simulink model "case9"  (R2024b)
settings: Solver=FixedStepAuto  StartTime=0  StopTime=1  FixedStep=1e-7  RelTol=1e-3
values from neighbouring files (symbols this model uses):
  SG_D_1_D = 0.01056    [IEEE9_case_parameters.m]    (also in case1_parameters.m; case2_parameters.m; case3_parameters.m; case4_parameters.m)
  SG_D_1_EnableSaturation = 0    [IEEE9_case_parameters.m]    (also in case1_parameters.m; case2_parameters.m; case3_parameters.m; case4_parameters.m)
  SG_D_1_f0 = 60    [IEEE9_case_parameters.m]    (also in case1_parameters.m; case2_parameters.m; case3_parameters.m; case4_parameters.m)
  SG_D_1_H = 7.5    [IEEE9_case_parameters.m]    (also in case1_parameters.m; case2_parameters.m; case3_parameters.m; case4_parameters.m)
  SG_D_1_K_A = 20    [IEEE9_case_parameters.m]    (also in case1_parameters.m; case2_parameters.m; case3_parameters.m; case4_parameters.m)
  SG_D_1_K_E = 1.000000e+1    (= 10)    [IEEE9_case_parameters.m]    (also in case1_parameters.m; case2_parameters.m; case3_parameters.m; case4_parameters.m)
  SG_D_1_K_F = 2.363    [IEEE9_case_parameters.m]    (also in case1_parameters.m; case2_parameters.m; case3_parameters.m; case4_parameters.m)
  SG_D_1_K_s = 0.5    [IEEE9_case_parameters.m]    (also in case1_parameters.m = 5; case2_parameters.m = 5; case3_parameters.m = 5; case4_parameters.m = 5)
  SG_D_1_R_a = 0.001088    [IEEE9_case_parameters.m]    (also in case1_parameters.m; case2_parameters.m; case3_parameters.m; case4_parameters.m)
  SG_D_1_S_A = 1    [IEEE9_case_parameters.m]    (also in case1_parameters.m; case2_parameters.m; case3_parameters.m; case4_parameters.m)
  SG_D_1_S_B = 0.103    [IEEE9_case_parameters.m]    (also in case1_parameters.m; case2_parameters.m; case3_parameters.m; case4_parameters.m)
  SG_D_1_S_N = 10.659857    [IEEE9_case_parameters.m]    (also in case1_parameters.m; case2_parameters.m; case3_parameters.m; case4_parameters.m)
  SG_D_1_SpeedPara = 200    [IEEE9_case_parameters.m]    (also in case1_parameters.m; case2_parameters.m; case3_parameters.m; case4_parameters.m)
  SG_D_1_T_0 = 0.720173    [IEEE9_case_parameters.m]    (also in case1_parameters.m = 0.755522; case2_parameters.m = 0.808931; case3_parameters.m = 0.869402; case4_parameters.m = 0.729316)
  SG_D_1_T_1 = 0.3    [IEEE9_case_parameters.m]    (also in case1_parameters.m; case2_parameters.m; case3_parameters.m; case4_parameters.m)
  SG_D_1_T_2 = 0.05    [IEEE9_case_parameters.m]    (also in case1_parameters.m; case2_parameters.m; case3_parameters.m; case4_parameters.m)
  SG_D_1_T_3 = 0.02    [IEEE9_case_parameters.m]    (also in case1_parameters.m; case2_parameters.m; case3_parameters.m; case4_parameters.m)
  SG_D_1_T_4 = 0.005    [IEEE9_case_parameters.m]    (also in case1_parameters.m; case2_parameters.m; case3_parameters.m; case4_parameters.m)
  SG_D_1_T_A = 0.02    [IEEE9_case_parameters.m]    (also in case1_parameters.m; case2_parameters.m; case3_parameters.m; case4_parameters.m)
  SG_D_1_T_dd = 8.000000e+0    (= 8)    [IEEE9_case_parameters.m]    (also in case1_parameters.m; case2_parameters.m; case3_parameters.m; case4_parameters.m)
  SG_D_1_T_ddd = 0.04    [IEEE9_case_parameters.m]    (also in case1_parameters.m; case2_parameters.m; case3_parameters.m; case4_parameters.m)
  SG_D_1_T_E = 0.314    [IEEE9_case_parameters.m]    (also in case1_parameters.m; case2_parameters.m; case3_parameters.m; case4_parameters.m)
  SG_D_1_T_F = 0.35    [IEEE9_case_parameters.m]    (also in case1_parameters.m; case2_parameters.m; case3_parameters.m; case4_parameters.m)
  SG_D_1_T_qd = 0.8    [IEEE9_case_parameters.m]    (also in case1_parameters.m; case2_parameters.m; case3_parameters.m; case4_parameters.m)
  SG_D_1_T_qdd = 0.02    [IEEE9_case_parameters.m]    (also in case1_parameters.m; case2_parameters.m; case3_parameters.m; case4_parameters.m)
  SG_D_1_T_speed = 0.1    [IEEE9_case_parameters.m]    (also in case1_parameters.m = 200; case2_parameters.m = 200; case3_parameters.m = 200; case4_parameters.m = 200)
  SG_D_1_T_w = 0.5    [IEEE9_case_parameters.m]    (also in case1_parameters.m; case2_parameters.m; case3_parameters.m; case4_parameters.m)
  SG_D_1_V_ref = 1.990276    [IEEE9_case_parameters.m]    (also in case1_parameters.m = 2.042296; case2_parameters.m = 2.051388; case3_parameters.m = 2.089584; case4_parameters.m = 2.01845)
  SG_D_1_w_ref = 376.991118    [IEEE9_case_parameters.m]    (also in case1_parameters.m; case2_parameters.m; case3_parameters.m; case4_parameters.m)
  SG_D_1_wb = 6.000000e+1    (= 60)    [IEEE9_case_parameters.m]    (also in case1_parameters.m; case2_parameters.m; case3_parameters.m; case4_parameters.m)
  SG_D_1_x_d = 1.9    [IEEE9_case_parameters.m]    (also in case1_parameters.m; case2_parameters.m; case3_parameters.m; case4_parameters.m)
  SG_D_1_x_dd = 0.302    [IEEE9_case_parameters.m]    (also in case1_parameters.m; case2_parameters.m; case3_parameters.m; case4_parameters.m)
  SG_D_1_x_ddd = 0.204    [IEEE9_case_parameters.m]    (also in case1_parameters.m; case2_parameters.m; case3_parameters.m; case4_parameters.m)
  SG_D_1_x_l = 0.05    [IEEE9_case_parameters.m]    (also in case1_parameters.m; case2_parameters.m; case3_parameters.m; case4_parameters.m)
  SG_D_1_x_q = 1.3    [IEEE9_case_parameters.m]    (also in case1_parameters.m; case2_parameters.m; case3_parameters.m; case4_parameters.m)
  SG_D_1_x_qd = 0.5    [IEEE9_case_parameters.m]    (also in case1_parameters.m; case2_parameters.m; case3_parameters.m; case4_parameters.m)
  SG_D_1_x_qdd = 0.3    [IEEE9_case_parameters.m]    (also in case1_parameters.m; case2_parameters.m; case3_parameters.m; case4_parameters.m)
  SG_D_2_D = 0.02    [IEEE9_case_parameters.m]    (also in case1_parameters.m; case2_parameters.m; case3_parameters.m; case4_parameters.m)
  SG_D_2_EnableSaturation = 0    [IEEE9_case_parameters.m]    (also in case1_parameters.m; case2_parameters.m; case3_parameters.m; case4_parameters.m)
  SG_D_2_f0 = 60    [IEEE9_case_parameters.m]    (also in case1_parameters.m; case2_parameters.m; case3_parameters.m; case4_parameters.m)
  SG_D_2_H = 8.000000e+0    (= 8)    [IEEE9_case_parameters.m]    (also in case1_parameters.m; case2_parameters.m; case3_parameters.m; case4_parameters.m)
  SG_D_2_K_A = 20    [IEEE9_case_parameters.m]    (also in case1_parameters.m; case2_parameters.m; case3_parameters.m; case4_parameters.m)
  SG_D_2_K_E = 1.000000e+1    (= 10)    [IEEE9_case_parameters.m]    (also in case1_parameters.m; case2_parameters.m; case3_parameters.m; case4_parameters.m)
  SG_D_2_K_F = 2.363    [IEEE9_case_parameters.m]    (also in case1_parameters.m; case2_parameters.m; case3_parameters.m; case4_parameters.m)
  SG_D_2_K_s = 0.5    [IEEE9_case_parameters.m]    (also in case1_parameters.m = 4; case2_parameters.m = 4; case3_parameters.m = 4; case4_parameters.m = 4)
  SG_D_2_R_a = 0.001088    [IEEE9_case_parameters.m]    (also in case1_parameters.m; case2_parameters.m; case3_parameters.m; case4_parameters.m)
  SG_D_2_S_A = 1    [IEEE9_case_parameters.m]    (also in case1_parameters.m; case2_parameters.m; case3_parameters.m; case4_parameters.m)
  SG_D_2_S_B = 0.103    [IEEE9_case_parameters.m]    (also in case1_parameters.m; case2_parameters.m; case3_parameters.m; case4_parameters.m)
  SG_D_2_S_N = 10.659857    [IEEE9_case_parameters.m]    (also in case1_parameters.m; case2_parameters.m; case3_parameters.m; case4_parameters.m)
  SG_D_2_SpeedPara = 200    [IEEE9_case_parameters.m]    (also in case1_parameters.m; case2_parameters.m; case3_parameters.m; case4_parameters.m)
  SG_D_2_T_0 = 1.632913    [IEEE9_case_parameters.m]    (also in case1_parameters.m = 1.632925; case2_parameters.m = 1.632915; case3_parameters.m = 1.632914; case4_parameters.m = 1.632927)
  SG_D_2_T_1 = 0.2    [IEEE9_case_parameters.m]    (also in case1_parameters.m; case2_parameters.m; case3_parameters.m; case4_parameters.m)
  SG_D_2_T_2 = 0.05    [IEEE9_case_parameters.m]    (also in case1_parameters.m; case2_parameters.m; case3_parameters.m; case4_parameters.m)
  SG_D_2_T_3 = 0.02    [IEEE9_case_parameters.m]    (also in case1_parameters.m; case2_parameters.m; case3_parameters.m; case4_parameters.m)
  SG_D_2_T_4 = 0.005    [IEEE9_case_parameters.m]    (also in case1_parameters.m; case2_parameters.m; case3_parameters.m; case4_parameters.m)
  SG_D_2_T_A = 0.02    [IEEE9_case_parameters.m]    (also in case1_parameters.m; case2_parameters.m; case3_parameters.m; case4_parameters.m)
  SG_D_2_T_dd = 7.9    [IEEE9_case_parameters.m]    (also in case1_parameters.m; case2_parameters.m; case3_parameters.m; case4_parameters.m)
  SG_D_2_T_ddd = 0.04    [IEEE9_case_parameters.m]    (also in case1_parameters.m; case2_parameters.m; case3_parameters.m; case4_parameters.m)
  SG_D_2_T_E = 0.314    [IEEE9_case_parameters.m]    (also in case1_parameters.m; case2_parameters.m; case3_parameters.m; case4_parameters.m)
  SG_D_2_T_F = 0.35    [IEEE9_case_parameters.m]    (also in case1_parameters.m; case2_parameters.m; case3_parameters.m; case4_parameters.m)
  SG_D_2_T_qd = 0.8    [IEEE9_case_parameters.m]    (also in case1_parameters.m; case2_parameters.m; case3_parameters.m; case4_parameters.m)
  SG_D_2_T_qdd = 0.015    [IEEE9_case_parameters.m]    (also in case1_parameters.m; case2_parameters.m; case3_parameters.m; case4_parameters.m)
  SG_D_2_T_speed = 0.1    [IEEE9_case_parameters.m]    (also in case1_parameters.m = 150; case2_parameters.m = 150; case3_parameters.m = 150; case4_parameters.m = 150)
  SG_D_2_T_w = 0.35    [IEEE9_case_parameters.m]    (also in case1_parameters.m; case2_parameters.m; case3_parameters.m; case4_parameters.m)
  SG_D_2_V_ref = 2.58547    [IEEE9_case_parameters.m]    (also in case1_parameters.m = 2.597896; case2_parameters.m = 2.587136; case3_parameters.m = 2.586042; case4_parameters.m = 2.599679)
  SG_D_2_w_ref = 376.991118    [IEEE9_case_parameters.m]    (also in case1_parameters.m; case2_parameters.m; case3_parameters.m; case4_parameters.m)
  SG_D_2_wb = 6.000000e+1    (= 60)    [IEEE9_case_parameters.m]    (also in case1_parameters.m; case2_parameters.m; case3_parameters.m; case4_parameters.m)
  SG_D_2_x_d = 1.8    [IEEE9_case_parameters.m]    (also in case1_parameters.m; case2_parameters.m; case3_parameters.m; case4_parameters.m)
  SG_D_2_x_dd = 0.302    [IEEE9_case_parameters.m]    (also in case1_parameters.m; case2_parameters.m; case3_parameters.m; case4_parameters.m)
  SG_D_2_x_ddd = 0.204    [IEEE9_case_parameters.m]    (also in case1_parameters.m; case2_parameters.m; case3_parameters.m; case4_parameters.m)
  SG_D_2_x_l = 0.05    [IEEE9_case_parameters.m]    (also in case1_parameters.m; case2_parameters.m; case3_parameters.m; case4_parameters.m)
  SG_D_2_x_q = 1.25    [IEEE9_case_parameters.m]    (also in case1_parameters.m; case2_parameters.m; case3_parameters.m; case4_parameters.m)
  SG_D_2_x_qd = 0.5    [IEEE9_case_parameters.m]    (also in case1_parameters.m; case2_parameters.m; case3_parameters.m; case4_parameters.m)
  SG_D_2_x_qdd = 0.3    [IEEE9_case_parameters.m]    (also in case1_parameters.m; case2_parameters.m; case3_parameters.m; case4_parameters.m)
  SG_D_3_D = 0.02    [IEEE9_case_parameters.m]    (also in case1_parameters.m; case2_parameters.m; case3_parameters.m; case4_parameters.m)
  SG_D_3_EnableSaturation = 0    [IEEE9_case_parameters.m]    (also in case1_parameters.m; case2_parameters.m; case3_parameters.m; case4_parameters.m)
  SG_D_3_f0 = 60    [IEEE9_case_parameters.m]    (also in case1_parameters.m; case2_parameters.m; case3_parameters.m; case4_parameters.m)
  SG_D_3_H = 7.7    [IEEE9_case_parameters.m]    (also in case1_parameters.m; case2_parameters.m; case3_parameters.m; case4_parameters.m)
  SG_D_3_K_A = 20    [IEEE9_case_parameters.m]    (also in case1_parameters.m; case2_parameters.m; case3_parameters.m; case4_parameters.m)
  SG_D_3_K_E = 1.000000e+1    (= 10)    [IEEE9_case_parameters.m]    (also in case1_parameters.m; case2_parameters.m; case3_parameters.m; case4_parameters.m)
  SG_D_3_K_F = 2.363    [IEEE9_case_parameters.m]    (also in case1_parameters.m; case2_parameters.m; case3_parameters.m; case4_parameters.m)
  SG_D_3_K_s = 0.2    [IEEE9_case_parameters.m]    (also in case1_parameters.m = 2; case2_parameters.m = 2; case3_parameters.m = 2; case4_parameters.m = 2)
  SG_D_3_R_a = 0.001088    [IEEE9_case_parameters.m]    (also in case1_parameters.m; case2_parameters.m; case3_parameters.m; case4_parameters.m)
  SG_D_3_S_A = 1    [IEEE9_case_parameters.m]    (also in case1_parameters.m; case2_parameters.m; case3_parameters.m; case4_parameters.m)
  SG_D_3_S_B = 0.103    [IEEE9_case_parameters.m]    (also in case1_parameters.m; case2_parameters.m; case3_parameters.m; case4_parameters.m)
  SG_D_3_S_N = 10.659857    [IEEE9_case_parameters.m]    (also in case1_parameters.m; case2_parameters.m; case3_parameters.m; case4_parameters.m)
  SG_D_3_SpeedPara = 200    [IEEE9_case_parameters.m]    (also in case1_parameters.m; case2_parameters.m; case3_parameters.m; case4_parameters.m)
  SG_D_3_T_0 = 0.850788    [IEEE9_case_parameters.m]    (also in case1_parameters.m = 0.850786; case2_parameters.m = 0.850787; case3_parameters.m; case4_parameters.m = 0.850786)
  SG_D_3_T_1 = 0.2    [IEEE9_case_parameters.m]    (also in case1_parameters.m; case2_parameters.m; case3_parameters.m; case4_parameters.m)
  SG_D_3_T_2 = 0.05    [IEEE9_case_parameters.m]    (also in case1_parameters.m; case2_parameters.m; case3_parameters.m; case4_parameters.m)
  SG_D_3_T_3 = 0.02    [IEEE9_case_parameters.m]    (also in case1_parameters.m; case2_parameters.m; case3_parameters.m; case4_parameters.m)
  SG_D_3_T_4 = 0.005    [IEEE9_case_parameters.m]    (also in case1_parameters.m; case2_parameters.m; case3_parameters.m; case4_parameters.m)
  SG_D_3_T_A = 0.02    [IEEE9_case_parameters.m]    (also in case1_parameters.m; case2_parameters.m; case3_parameters.m; case4_parameters.m)
  SG_D_3_T_dd = 8.1    [IEEE9_case_parameters.m]    (also in case1_parameters.m; case2_parameters.m; case3_parameters.m; case4_parameters.m)
  SG_D_3_T_ddd = 0.04    [IEEE9_case_parameters.m]    (also in case1_parameters.m; case2_parameters.m; case3_parameters.m; case4_parameters.m)
  SG_D_3_T_E = 0.314    [IEEE9_case_parameters.m]    (also in case1_parameters.m; case2_parameters.m; case3_parameters.m; case4_parameters.m)
  SG_D_3_T_F = 0.35    [IEEE9_case_parameters.m]    (also in case1_parameters.m; case2_parameters.m; case3_parameters.m; case4_parameters.m)
  SG_D_3_T_qd = 0.8    [IEEE9_case_parameters.m]    (also in case1_parameters.m; case2_parameters.m; case3_parameters.m; case4_parameters.m)
  SG_D_3_T_qdd = 0.015    [IEEE9_case_parameters.m]    (also in case1_parameters.m; case2_parameters.m; case3_parameters.m; case4_parameters.m)
  SG_D_3_T_speed = 0.1    [IEEE9_case_parameters.m]    (also in case1_parameters.m = 180; case2_parameters.m = 180; case3_parameters.m = 180; case4_parameters.m = 180)
  SG_D_3_T_w = 0.4    [IEEE9_case_parameters.m]    (also in case1_parameters.m; case2_parameters.m; case3_parameters.m; case4_parameters.m)
  SG_D_3_V_ref = 1.892727    [IEEE9_case_parameters.m]    (also in case1_parameters.m = 1.906439; case2_parameters.m = 1.895535; case3_parameters.m = 1.892105; case4_parameters.m = 1.906598)
  SG_D_3_w_ref = 376.991118    [IEEE9_case_parameters.m]    (also in case1_parameters.m; case2_parameters.m; case3_parameters.m; case4_parameters.m)
  SG_D_3_wb = 6.000000e+1    (= 60)    [IEEE9_case_parameters.m]    (also in case1_parameters.m; case2_parameters.m; case3_parameters.m; case4_parameters.m)
  SG_D_3_x_d = 1.85    [IEEE9_case_parameters.m]    (also in case1_parameters.m; case2_parameters.m; case3_parameters.m; case4_parameters.m)
  SG_D_3_x_dd = 0.302    [IEEE9_case_parameters.m]    (also in case1_parameters.m; case2_parameters.m; case3_parameters.m; case4_parameters.m)
  SG_D_3_x_ddd = 0.204    [IEEE9_case_parameters.m]    (also in case1_parameters.m; case2_parameters.m; case3_parameters.m; case4_parameters.m)
  SG_D_3_x_l = 0.05    [IEEE9_case_parameters.m]    (also in case1_parameters.m; case2_parameters.m; case3_parameters.m; case4_parameters.m)
  SG_D_3_x_q = 1.2    [IEEE9_case_parameters.m]    (also in case1_parameters.m; case2_parameters.m; case3_parameters.m; case4_parameters.m)
  SG_D_3_x_qd = 0.5    [IEEE9_case_parameters.m]    (also in case1_parameters.m; case2_parameters.m; case3_parameters.m; case4_parameters.m)
  SG_D_3_x_qdd = 0.3    [IEEE9_case_parameters.m]    (also in case1_parameters.m; case2_parameters.m; case3_parameters.m; case4_parameters.m)
(part 3 of 12)

== system case9/AC_1/d_vq_bus_2_block ==
  note: d_vq_bus_2 in case9
      | $37699111.8430775\,\mathrm{iq}_{\mathrm{bus},2}-376.991118430775\,\mathrm{vd}_{\mathrm{bus},2}$
      | Automatically generated on 2025-10-31 19:35:33 .
  Alge_iq_bus_2_77b03 : Inport
  State_vd_bus_2_31c31 : Inport  Port=2
  Constant_376.991118430775_297b4 : Constant  Value=376.991118430775
  Constant_37699111.8430775_23c38 : Constant  Value=37699111.8430775
  Product_78845 : Product
  Product_c8408 : Product
  Subtract_e18ad : Sum  Inputs=+-
  Blockout_d_vq_bus_2_4c26a : Outport
  wires:
  Constant_37699111.8430775_23c38/1 -> Product_78845/1
  Constant_376.991118430775_297b4/1 -> Product_c8408/1
  Alge_iq_bus_2_77b03/1 -> Product_78845/2
  State_vd_bus_2_31c31/1 -> Product_c8408/2
  Product_78845/1 -> Subtract_e18ad/1
  Product_c8408/1 -> Subtract_e18ad/2
  Subtract_e18ad/1 -> Blockout_d_vq_bus_2_4c26a/1

== system case9/AC_1/d_vq_bus_3_block ==
  note: d_vq_bus_3 in case9
      | $37699111.8430775\,\mathrm{iq}_{\mathrm{bus},3}-376.991118430775\,\mathrm{vd}_{\mathrm{bus},3}$
      | Automatically generated on 2025-10-31 19:35:34 .
  Alge_iq_bus_3_cc23e : Inport
  State_vd_bus_3_6cfca : Inport  Port=2
  Constant_376.991118430775_aad21 : Constant  Value=376.991118430775
  Constant_37699111.8430775_489f0 : Constant  Value=37699111.8430775
  Product_2d405 : Product
  Product_442e1 : Product
  Subtract_58085 : Sum  Inputs=+-
  Blockout_d_vq_bus_3_a4433 : Outport
  wires:
  Constant_37699111.8430775_489f0/1 -> Product_2d405/1
  Constant_376.991118430775_aad21/1 -> Product_442e1/1
  Alge_iq_bus_3_cc23e/1 -> Product_2d405/2
  State_vd_bus_3_6cfca/1 -> Product_442e1/2
  Product_2d405/1 -> Subtract_58085/1
  Product_442e1/1 -> Subtract_58085/2
  Subtract_58085/1 -> Blockout_d_vq_bus_3_a4433/1

== system case9/AC_1/d_vq_bus_4_block ==
  note: d_vq_bus_4 in case9
      | $2257.43184689087\,\mathrm{iq}_{\mathrm{bus},4}-376.991118430775\,\mathrm{vd}_{\mathrm{bus},4}$
      | Automatically generated on 2025-10-31 19:35:34 .
  Alge_iq_bus_4_57fc4 : Inport
  State_vd_bus_4_4807b : Inport  Port=2
  Constant_2257.43184689087_35413 : Constant  Value=2257.43184689087
  Constant_376.991118430775_cfbfc : Constant  Value=376.991118430775
  Product_cb25e : Product
  Product_f6559 : Product
  Subtract_ca4f2 : Sum  Inputs=+-
  Blockout_d_vq_bus_4_b4e62 : Outport
  wires:
  Constant_2257.43184689087_35413/1 -> Product_f6559/1
  Constant_376.991118430775_cfbfc/1 -> Product_cb25e/1
  Alge_iq_bus_4_57fc4/1 -> Product_f6559/2
  State_vd_bus_4_4807b/1 -> Product_cb25e/2
  Product_f6559/1 -> Subtract_ca4f2/1
  Product_cb25e/1 -> Subtract_ca4f2/2
  Subtract_ca4f2/1 -> Blockout_d_vq_bus_4_b4e62/1

== system case9/AC_1/d_vq_bus_5_block ==
  note: d_vq_bus_5 in case9
      | $1461.2058853906\,\mathrm{iq}_{\mathrm{bus},5}-376.991118430775\,\mathrm{vd}_{\mathrm{bus},5}$
      | Automatically generated on 2025-10-31 19:35:35 .
  Alge_iq_bus_5_8c66c : Inport
  State_vd_bus_5_846f7 : Inport  Port=2
  Constant_1461.2058853906_0d7a9 : Constant  Value=1461.2058853906
  Constant_376.991118430775_e6df8 : Constant  Value=376.991118430775
  Product_c1e2f : Product
  Product_fd608 : Product
  Subtract_c2c85 : Sum  Inputs=+-
  Blockout_d_vq_bus_5_0bbb7 : Outport
  wires:
  Constant_1461.2058853906_0d7a9/1 -> Product_fd608/1
  Constant_376.991118430775_e6df8/1 -> Product_c1e2f/1
  Alge_iq_bus_5_8c66c/1 -> Product_fd608/2
  State_vd_bus_5_846f7/1 -> Product_c1e2f/2
  Product_fd608/1 -> Subtract_c2c85/1
  Product_c1e2f/1 -> Subtract_c2c85/2
  Subtract_c2c85/1 -> Blockout_d_vq_bus_5_0bbb7/1

== system case9/AC_1/d_vq_bus_6_block ==
  note: d_vq_bus_6 in case9
      | $1329.77466818616\,\mathrm{iq}_{\mathrm{bus},6}-376.991118430775\,\mathrm{vd}_{\mathrm{bus},6}$
      | Automatically generated on 2025-10-31 19:35:35 .
  Alge_iq_bus_6_d852c : Inport
  State_vd_bus_6_933d9 : Inport  Port=2
  Constant_1329.77466818616_4ee96 : Constant  Value=1329.77466818616
  Constant_376.991118430775_b81da : Constant  Value=376.991118430775
  Product_b7a54 : Product
  Product_c8743 : Product
  Subtract_aadba : Sum  Inputs=+-
  Blockout_d_vq_bus_6_9d5e1 : Outport
  wires:
  Constant_1329.77466818616_4ee96/1 -> Product_c8743/1
  Constant_376.991118430775_b81da/1 -> Product_b7a54/1
  Alge_iq_bus_6_d852c/1 -> Product_c8743/2
  State_vd_bus_6_933d9/1 -> Product_b7a54/2
  Product_c8743/1 -> Subtract_aadba/1
  Product_b7a54/1 -> Subtract_aadba/2
  Subtract_aadba/1 -> Blockout_d_vq_bus_6_9d5e1/1

== system case9/AC_1/d_vq_bus_7_block ==
  note: d_vq_bus_7 in case9
      | $2106.09563369148\,\mathrm{iq}_{\mathrm{bus},7}-376.991118430775\,\mathrm{vd}_{\mathrm{bus},7}$
      | Automatically generated on 2025-10-31 19:35:36 .
  Alge_iq_bus_7_10ac4 : Inport
  State_vd_bus_7_f1873 : Inport  Port=2
  Constant_2106.09563369148_b1513 : Constant  Value=2106.09563369148
  Constant_376.991118430775_e1123 : Constant  Value=376.991118430775
  Product_6b0d5 : Product
  Product_fc3db : Product
  Subtract_4ac9d : Sum  Inputs=+-
  Blockout_d_vq_bus_7_bd4da : Outport
  wires:
  Constant_2106.09563369148_b1513/1 -> Product_fc3db/1
  Product_6b0d5/1 -> Subtract_4ac9d/2
  Alge_iq_bus_7_10ac4/1 -> Product_fc3db/2
  Constant_376.991118430775_e1123/1 -> Product_6b0d5/1
  Subtract_4ac9d/1 -> Blockout_d_vq_bus_7_bd4da/1
  State_vd_bus_7_f1873/1 -> Product_6b0d5/2
  Product_fc3db/1 -> Subtract_4ac9d/1

== system case9/AC_1/d_vq_bus_8_block ==
  note: d_vq_bus_8 in case9
      | $1657.10381727813\,\mathrm{iq}_{\mathrm{bus},8}-376.991118430775\,\mathrm{vd}_{\mathrm{bus},8}$
      | Automatically generated on 2025-10-31 19:35:36 .
  Alge_iq_bus_8_70786 : Inport
  State_vd_bus_8_2f4e8 : Inport  Port=2
  Constant_1657.10381727813_470a7 : Constant  Value=1657.10381727813
  Constant_376.991118430775_75430 : Constant  Value=376.991118430775
  Product_04e24 : Product
  Product_0a383 : Product
  Subtract_4f591 : Sum  Inputs=+-
  Blockout_d_vq_bus_8_7a639 : Outport
  wires:
  Constant_1657.10381727813_470a7/1 -> Product_04e24/1
  Constant_376.991118430775_75430/1 -> Product_0a383/1
  Alge_iq_bus_8_70786/1 -> Product_04e24/2
  State_vd_bus_8_2f4e8/1 -> Product_0a383/2
  Product_04e24/1 -> Subtract_4f591/1
  Product_0a383/1 -> Subtract_4f591/2
  Subtract_4f591/1 -> Blockout_d_vq_bus_8_7a639/1

== system case9/AC_1/d_vq_bus_9_block ==
  note: d_vq_bus_9 in case9
      | $1564.27849971276\,\mathrm{iq}_{\mathrm{bus},9}-376.991118430775\,\mathrm{vd}_{\mathrm{bus},9}$
      | Automatically generated on 2025-10-31 19:35:37 .
  Alge_iq_bus_9_d89c6 : Inport
  State_vd_bus_9_9eb2e : Inport  Port=2
  Constant_1564.27849971276_ed724 : Constant  Value=1564.27849971276
  Constant_376.991118430775_3314c : Constant  Value=376.991118430775
  Product_29196 : Product
  Product_ab7b2 : Product
  Subtract_c7e30 : Sum  Inputs=+-
  Blockout_d_vq_bus_9_68009 : Outport
  wires:
  Constant_1564.27849971276_ed724/1 -> Product_29196/1
  Constant_376.991118430775_3314c/1 -> Product_ab7b2/1
  Alge_iq_bus_9_d89c6/1 -> Product_29196/2
  State_vd_bus_9_9eb2e/1 -> Product_ab7b2/2
  Product_29196/1 -> Subtract_c7e30/1
  Product_ab7b2/1 -> Subtract_c7e30/2
  Subtract_c7e30/1 -> Blockout_d_vq_bus_9_68009/1

== system case9/AC_1/id_bus_1_block ==
  note: id_bus_1 in case9
      | $\mathrm{id}_{\mathrm{SG},D,1}-\mathrm{id}_{\mathrm{line},1,4}$
      | Automatically generated on 2025-10-31 19:35:48 .
  Input_id_SG_D_1_08570 : Inport
  State_id_line_1_4_a7c42 : Inport  Port=2
  Subtract_91534 : Sum  Inputs=+-
  Blockout_id_bus_1_e658d : Outport
  wires:
  Input_id_SG_D_1_08570/1 -> Subtract_91534/1
  State_id_line_1_4_a7c42/1 -> Subtract_91534/2
  Subtract_91534/1 -> Blockout_id_bus_1_e658d/1

== system case9/AC_1/id_bus_2_block ==
  note: id_bus_2 in case9
      | $\mathrm{id}_{\mathrm{SG},D,2}+\mathrm{id}_{\mathrm{line},8,2}$
      | Automatically generated on 2025-10-31 19:35:49 .
  Input_id_SG_D_2_88308 : Inport
  State_id_line_8_2_4faa5 : Inport  Port=2
  Add_03b43 : Sum
  Blockout_id_bus_2_4fbc8 : Outport
  wires:
  Input_id_SG_D_2_88308/1 -> Add_03b43/1
  State_id_line_8_2_4faa5/1 -> Add_03b43/2
  Add_03b43/1 -> Blockout_id_bus_2_4fbc8/1

== system case9/AC_1/id_bus_3_block ==
  note: id_bus_3 in case9
      | $\mathrm{id}_{\mathrm{SG},D,3}-\mathrm{id}_{\mathrm{line},3,6}$
      | Automatically generated on 2025-10-31 19:35:50 .
  Input_id_SG_D_3_5e5e9 : Inport
  State_id_line_3_6_41fe6 : Inport  Port=2
  Subtract_f08cd : Sum  Inputs=+-
  Blockout_id_bus_3_b7ff3 : Outport
  wires:
  Input_id_SG_D_3_5e5e9/1 -> Subtract_f08cd/1
  State_id_line_3_6_41fe6/1 -> Subtract_f08cd/2
  Subtract_f08cd/1 -> Blockout_id_bus_3_b7ff3/1

== system case9/AC_1/id_bus_4_block ==
  note: id_bus_4 in case9
      | $\mathrm{id}_{\mathrm{line},1,4}-\mathrm{id}_{\mathrm{line},4,5}+\mathrm{id}_{\mathrm{line},9,4}$
      | Automatically generated on 2025-10-31 19:35:50 .
  State_id_line_1_4_cc172 : Inport
  State_id_line_4_5_e9164 : Inport  Port=2
  State_id_line_9_4_5b567 : Inport  Port=3
  Add_a2397 : Sum
  Subtract_6347f : Sum  Inputs=+-
  Blockout_id_bus_4_24f5c : Outport
  wires:
  State_id_line_9_4_5b567/1 -> Add_a2397/2
  State_id_line_1_4_cc172/1 -> Subtract_6347f/1
  State_id_line_4_5_e9164/1 -> Subtract_6347f/2
  Subtract_6347f/1 -> Add_a2397/1
  Add_a2397/1 -> Blockout_id_bus_4_24f5c/1

== system case9/AC_1/id_bus_5_block ==
  note: id_bus_5 in case9
      | $\mathrm{id}_{\mathrm{line},4,5}-\mathrm{id}_{\mathrm{load},5}-\mathrm{id}_{\mathrm{line},5,6}$
      | Automatically generated on 2025-10-31 19:35:51 .
  State_id_load_5_eb383 : Inport
  State_id_line_4_5_62aa2 : Inport  Port=2
  State_id_line_5_6_da129 : Inport  Port=3
  Add_6d8ca : Sum
  Constant_-1_b7f07 : Constant  Value=-1
  Product_f9331 : Product
  Subtract_12f77 : Sum  Inputs=+-
  Blockout_id_bus_5_f01f3 : Outport
  wires:
  Subtract_12f77/1 -> Blockout_id_bus_5_f01f3/1
  State_id_line_4_5_62aa2/1 -> Add_6d8ca/2
  Constant_-1_b7f07/1 -> Product_f9331/1
  Add_6d8ca/1 -> Subtract_12f77/1
  State_id_load_5_eb383/1 -> Product_f9331/2
  Product_f9331/1 -> Add_6d8ca/1
  State_id_line_5_6_da129/1 -> Subtract_12f77/2

== system case9/AC_1/id_bus_6_block ==
  note: id_bus_6 in case9
      | $\mathrm{id}_{\mathrm{line},3,6}+\mathrm{id}_{\mathrm{line},5,6}-\mathrm{id}_{\mathrm{line},6,7}$
      | Automatically generated on 2025-10-31 19:35:51 .
  State_id_line_3_6_98865 : Inport
  State_id_line_5_6_ca554 : Inport  Port=2
  State_id_line_6_7_45885 : Inport  Port=3
  Add_ff3d5 : Sum
  Subtract_af532 : Sum  Inputs=+-
  Blockout_id_bus_6_9161d : Outport
  wires:
  State_id_line_6_7_45885/1 -> Subtract_af532/2
  State_id_line_3_6_98865/1 -> Add_ff3d5/1
  State_id_line_5_6_ca554/1 -> Add_ff3d5/2
  Add_ff3d5/1 -> Subtract_af532/1
  Subtract_af532/1 -> Blockout_id_bus_6_9161d/1

== system case9/AC_1/id_bus_7_block ==
  note: id_bus_7 in case9
      | $\mathrm{id}_{\mathrm{line},6,7}-\mathrm{id}_{\mathrm{load},7}-\mathrm{id}_{\mathrm{line},7,8}$
      | Automatically generated on 2025-10-31 19:35:52 .
  State_id_load_7_63198 : Inport
  State_id_line_6_7_cc3af : Inport  Port=2
  State_id_line_7_8_e44d5 : Inport  Port=3
  Add_0a43a : Sum
  Constant_-1_d528d : Constant  Value=-1
  Product_cca70 : Product
  Subtract_121d7 : Sum  Inputs=+-
  Blockout_id_bus_7_7b061 : Outport
  wires:
  Subtract_121d7/1 -> Blockout_id_bus_7_7b061/1
  State_id_line_6_7_cc3af/1 -> Add_0a43a/2
  Constant_-1_d528d/1 -> Product_cca70/1
  Add_0a43a/1 -> Subtract_121d7/1
  State_id_load_7_63198/1 -> Product_cca70/2
  Product_cca70/1 -> Add_0a43a/1
  State_id_line_7_8_e44d5/1 -> Subtract_121d7/2

== system case9/AC_1/id_bus_8_block ==
  note: id_bus_8 in case9
      | $\mathrm{id}_{\mathrm{line},7,8}-\mathrm{id}_{\mathrm{line},8,2}-\mathrm{id}_{\mathrm{line},8,9}$
      | Automatically generated on 2025-10-31 19:35:52 .
  State_id_line_7_8_c3e2c : Inport
  State_id_line_8_2_a7a20 : Inport  Port=2
  State_id_line_8_9_eb516 : Inport  Port=3
  Subtract_81ee0 : Sum  Inputs=+-
  Subtract_90e76 : Sum  Inputs=+-
  Blockout_id_bus_8_5999e : Outport
  wires:
  State_id_line_8_9_eb516/1 -> Subtract_90e76/2
  State_id_line_7_8_c3e2c/1 -> Subtract_81ee0/1
  State_id_line_8_2_a7a20/1 -> Subtract_81ee0/2
  Subtract_81ee0/1 -> Subtract_90e76/1
  Subtract_90e76/1 -> Blockout_id_bus_8_5999e/1

== system case9/AC_1/id_bus_9_block ==
  note: id_bus_9 in case9
      | $\mathrm{id}_{\mathrm{line},8,9}-\mathrm{id}_{\mathrm{load},9}-\mathrm{id}_{\mathrm{line},9,4}$
      | Automatically generated on 2025-10-31 19:35:53 .
  State_id_load_9_75b19 : Inport
  State_id_line_8_9_b4415 : Inport  Port=2
  State_id_line_9_4_0707e : Inport  Port=3
  Add_57bd4 : Sum
  Constant_-1_9b138 : Constant  Value=-1
  Product_b75d7 : Product
  Subtract_90a28 : Sum  Inputs=+-
  Blockout_id_bus_9_2b9f8 : Outport
  wires:
  Subtract_90a28/1 -> Blockout_id_bus_9_2b9f8/1
  State_id_line_8_9_b4415/1 -> Add_57bd4/2
  Constant_-1_9b138/1 -> Product_b75d7/1
  Add_57bd4/1 -> Subtract_90a28/1
  State_id_load_9_75b19/1 -> Product_b75d7/2
  Product_b75d7/1 -> Add_57bd4/1
  State_id_line_9_4_0707e/1 -> Subtract_90a28/2

== system case9/AC_1/iq_bus_1_block ==
  note: iq_bus_1 in case9
      | $\mathrm{iq}_{\mathrm{SG},D,1}-\mathrm{iq}_{\mathrm{line},1,4}$
      | Automatically generated on 2025-10-31 19:35:48 .
  Input_iq_SG_D_1_4e7e5 : Inport
  State_iq_line_1_4_643e1 : Inport  Port=2
  Subtract_0b7e1 : Sum  Inputs=+-
  Blockout_iq_bus_1_d5df9 : Outport
  wires:
  Input_iq_SG_D_1_4e7e5/1 -> Subtract_0b7e1/1
  State_iq_line_1_4_643e1/1 -> Subtract_0b7e1/2
  Subtract_0b7e1/1 -> Blockout_iq_bus_1_d5df9/1

== system case9/AC_1/iq_bus_2_block ==
  note: iq_bus_2 in case9
      | $\mathrm{iq}_{\mathrm{SG},D,2}+\mathrm{iq}_{\mathrm{line},8,2}$
      | Automatically generated on 2025-10-31 19:35:49 .
  Input_iq_SG_D_2_07d64 : Inport
  State_iq_line_8_2_c72a6 : Inport  Port=2
  Add_6f1e2 : Sum
  Blockout_iq_bus_2_a9312 : Outport
  wires:
  Input_iq_SG_D_2_07d64/1 -> Add_6f1e2/1
  State_iq_line_8_2_c72a6/1 -> Add_6f1e2/2
  Add_6f1e2/1 -> Blockout_iq_bus_2_a9312/1

== system case9/AC_1/iq_bus_3_block ==
  note: iq_bus_3 in case9
      | $\mathrm{iq}_{\mathrm{SG},D,3}-\mathrm{iq}_{\mathrm{line},3,6}$
      | Automatically generated on 2025-10-31 19:35:50 .
  Input_iq_SG_D_3_3d9a6 : Inport
  State_iq_line_3_6_e1477 : Inport  Port=2
  Subtract_cf636 : Sum  Inputs=+-
  Blockout_iq_bus_3_d80df : Outport
  wires:
  Input_iq_SG_D_3_3d9a6/1 -> Subtract_cf636/1
  State_iq_line_3_6_e1477/1 -> Subtract_cf636/2
  Subtract_cf636/1 -> Blockout_iq_bus_3_d80df/1

== system case9/AC_1/iq_bus_4_block ==
  note: iq_bus_4 in case9
      | $\mathrm{iq}_{\mathrm{line},1,4}-\mathrm{iq}_{\mathrm{line},4,5}+\mathrm{iq}_{\mathrm{line},9,4}$
      | Automatically generated on 2025-10-31 19:35:50 .
  State_iq_line_1_4_0500a : Inport
  State_iq_line_4_5_fdcfc : Inport  Port=2
  State_iq_line_9_4_5dba6 : Inport  Port=3
  Add_2cb8a : Sum
  Subtract_12a1c : Sum  Inputs=+-
  Blockout_iq_bus_4_63b2e : Outport
  wires:
  State_iq_line_1_4_0500a/1 -> Subtract_12a1c/1
  State_iq_line_4_5_fdcfc/1 -> Subtract_12a1c/2
  Subtract_12a1c/1 -> Add_2cb8a/1
  State_iq_line_9_4_5dba6/1 -> Add_2cb8a/2
  Add_2cb8a/1 -> Blockout_iq_bus_4_63b2e/1

== system case9/AC_1/iq_bus_5_block ==
  note: iq_bus_5 in case9
      | $\mathrm{iq}_{\mathrm{line},4,5}-\mathrm{iq}_{\mathrm{load},5}-\mathrm{iq}_{\mathrm{line},5,6}$
      | Automatically generated on 2025-10-31 19:35:51 .
  State_iq_load_5_53083 : Inport
  State_iq_line_4_5_1b735 : Inport  Port=2
  State_iq_line_5_6_ad611 : Inport  Port=3
  Add_8b9b6 : Sum
  Constant_-1_bb83a : Constant  Value=-1
  Product_a4077 : Product
  Subtract_a4cd7 : Sum  Inputs=+-
  Blockout_iq_bus_5_6d5f4 : Outport
  wires:
  Subtract_a4cd7/1 -> Blockout_iq_bus_5_6d5f4/1
  State_iq_line_4_5_1b735/1 -> Add_8b9b6/2
  Constant_-1_bb83a/1 -> Product_a4077/1
  State_iq_load_5_53083/1 -> Product_a4077/2
  Product_a4077/1 -> Add_8b9b6/1
  Add_8b9b6/1 -> Subtract_a4cd7/1
  State_iq_line_5_6_ad611/1 -> Subtract_a4cd7/2

== system case9/AC_1/iq_bus_6_block ==
  note: iq_bus_6 in case9
      | $\mathrm{iq}_{\mathrm{line},3,6}+\mathrm{iq}_{\mathrm{line},5,6}-\mathrm{iq}_{\mathrm{line},6,7}$
      | Automatically generated on 2025-10-31 19:35:51 .
  State_iq_line_3_6_f0e75 : Inport
  State_iq_line_5_6_e5890 : Inport  Port=2
  State_iq_line_6_7_dc0b6 : Inport  Port=3
  Add_bc52c : Sum
  Subtract_56569 : Sum  Inputs=+-
  Blockout_iq_bus_6_68831 : Outport
  wires:
  State_iq_line_3_6_f0e75/1 -> Add_bc52c/1
  State_iq_line_5_6_e5890/1 -> Add_bc52c/2
  Add_bc52c/1 -> Subtract_56569/1
  State_iq_line_6_7_dc0b6/1 -> Subtract_56569/2
  Subtract_56569/1 -> Blockout_iq_bus_6_68831/1

== system case9/AC_1/iq_bus_7_block ==
  note: iq_bus_7 in case9
      | $\mathrm{iq}_{\mathrm{line},6,7}-\mathrm{iq}_{\mathrm{load},7}-\mathrm{iq}_{\mathrm{line},7,8}$
      | Automatically generated on 2025-10-31 19:35:52 .
  State_iq_load_7_bb003 : Inport
  State_iq_line_6_7_3541c : Inport  Port=2
  State_iq_line_7_8_7cd8b : Inport  Port=3
  Add_38c70 : Sum
  Constant_-1_cb640 : Constant  Value=-1
  Product_b0f0c : Product
  Subtract_2befd : Sum  Inputs=+-
  Blockout_iq_bus_7_79b7d : Outport
  wires:
  Subtract_2befd/1 -> Blockout_iq_bus_7_79b7d/1
  State_iq_line_6_7_3541c/1 -> Add_38c70/2
  Constant_-1_cb640/1 -> Product_b0f0c/1
  State_iq_load_7_bb003/1 -> Product_b0f0c/2
  Product_b0f0c/1 -> Add_38c70/1
  Add_38c70/1 -> Subtract_2befd/1
  State_iq_line_7_8_7cd8b/1 -> Subtract_2befd/2

== system case9/AC_1/iq_bus_8_block ==
  note: iq_bus_8 in case9
      | $\mathrm{iq}_{\mathrm{line},7,8}-\mathrm{iq}_{\mathrm{line},8,2}-\mathrm{iq}_{\mathrm{line},8,9}$
      | Automatically generated on 2025-10-31 19:35:52 .
  State_iq_line_7_8_eb6ae : Inport
  State_iq_line_8_2_645e0 : Inport  Port=2
  State_iq_line_8_9_a06f9 : Inport  Port=3
  Subtract_6178c : Sum  Inputs=+-
  Subtract_805af : Sum  Inputs=+-
  Blockout_iq_bus_8_ea31f : Outport
  wires:
  State_iq_line_7_8_eb6ae/1 -> Subtract_6178c/1
  State_iq_line_8_2_645e0/1 -> Subtract_6178c/2
  Subtract_6178c/1 -> Subtract_805af/1
  State_iq_line_8_9_a06f9/1 -> Subtract_805af/2
  Subtract_805af/1 -> Blockout_iq_bus_8_ea31f/1

== system case9/AC_1/iq_bus_9_block ==
  note: iq_bus_9 in case9
      | $\mathrm{iq}_{\mathrm{line},8,9}-\mathrm{iq}_{\mathrm{load},9}-\mathrm{iq}_{\mathrm{line},9,4}$
      | Automatically generated on 2025-10-31 19:35:53 .
  State_iq_load_9_8900a : Inport
  State_iq_line_8_9_87f07 : Inport  Port=2
  State_iq_line_9_4_4804a : Inport  Port=3
  Add_59aa3 : Sum
  Constant_-1_d5737 : Constant  Value=-1
  Product_5ef53 : Product
  Subtract_e189a : Sum  Inputs=+-
  Blockout_iq_bus_9_35f70 : Outport
  wires:
  Subtract_e189a/1 -> Blockout_iq_bus_9_35f70/1
  State_iq_line_8_9_87f07/1 -> Add_59aa3/2
  Constant_-1_d5737/1 -> Product_5ef53/1
  State_iq_load_9_8900a/1 -> Product_5ef53/2
  Product_5ef53/1 -> Add_59aa3/1
  Add_59aa3/1 -> Subtract_e189a/1
  State_iq_line_9_4_4804a/1 -> Subtract_e189a/2

== system case9/AC_1/vd_bus_1_out_block ==
  note: vd_bus_1_out in case9
      | $\mathrm{vd}_{\mathrm{bus},1}$
      | Automatically generated on 2025-10-31 19:35:48 .
  State_vd_bus_1_7b6a9 : Inport
  Blockout_vd_bus_1_out_57e40 : Outport
  wires:
  State_vd_bus_1_7b6a9/1 -> Blockout_vd_bus_1_out_57e40/1

== system case9/AC_1/vd_bus_2_out_block ==
  note: vd_bus_2_out in case9
      | $\mathrm{vd}_{\mathrm{bus},2}$
      | Automatically generated on 2025-10-31 19:35:48 .
  State_vd_bus_2_c52cc : Inport
  Blockout_vd_bus_2_out_204c7 : Outport
  wires:
  State_vd_bus_2_c52cc/1 -> Blockout_vd_bus_2_out_204c7/1

== system case9/AC_1/vd_bus_3_out_block ==
  note: vd_bus_3_out in case9
      | $\mathrm{vd}_{\mathrm{bus},3}$
      | Automatically generated on 2025-10-31 19:35:49 .
  State_vd_bus_3_a5a57 : Inport
  Blockout_vd_bus_3_out_0fd0d : Outport
  wires:
  State_vd_bus_3_a5a57/1 -> Blockout_vd_bus_3_out_0fd0d/1

== system case9/AC_1/vq_bus_1_out_block ==
  note: vq_bus_1_out in case9
      | $\mathrm{vq}_{\mathrm{bus},1}$
      | Automatically generated on 2025-10-31 19:35:48 .
  State_vq_bus_1_621b2 : Inport
  Blockout_vq_bus_1_out_92f46 : Outport
  wires:
  State_vq_bus_1_621b2/1 -> Blockout_vq_bus_1_out_92f46/1

== system case9/AC_1/vq_bus_2_out_block ==
  note: vq_bus_2_out in case9
      | $\mathrm{vq}_{\mathrm{bus},2}$
      | Automatically generated on 2025-10-31 19:35:48 .
  State_vq_bus_2_d267d : Inport
  Blockout_vq_bus_2_out_d1306 : Outport
  wires:
  State_vq_bus_2_d267d/1 -> Blockout_vq_bus_2_out_d1306/1

== system case9/AC_1/vq_bus_3_out_block ==
  note: vq_bus_3_out in case9
      | $\mathrm{vq}_{\mathrm{bus},3}$
      | Automatically generated on 2025-10-31 19:35:49 .
  State_vq_bus_3_04fbf : Inport
  Blockout_vq_bus_3_out_26b2e : Outport
  wires:
  State_vq_bus_3_04fbf/1 -> Blockout_vq_bus_3_out_26b2e/1

== system case9/Apparatus/SG_D_1 ==
  v_d_SG_D_1 : Inport
  v_q_SG_D_1 : Inport  Port=2
  E_fd_SG_D_1 : Integrator  InitialCondition=2.1681510267996753
  Px_1_SG_D_1 : Integrator  InitialCondition=0.0
  Px_2_SG_D_1 : Integrator  InitialCondition=0.0
  Px_3_SG_D_1 : Integrator  InitialCondition=-4.041451642418766e-30
  R_f_SG_D_1 : Integrator  InitialCondition=14.638116789507523
  T_e_SG_D_1_block : Subsystem
  T_m_SG_D_1 : Integrator  InitialCondition=0.8781809876188345
  V_f_SG_D_1 : Integrator  InitialCondition=21.681510267996753
  d_E_fd_SG_D_1_block : Subsystem
  d_Px_1_SG_D_1_block : Subsystem
  d_Px_2_SG_D_1_block : Subsystem
  d_Px_3_SG_D_1_block : Subsystem
  d_R_f_SG_D_1_block : Subsystem
  d_T_m_SG_D_1_block : Subsystem
  d_V_f_SG_D_1_block : Subsystem
  d_psi_1d_SG_D_1_block : Subsystem
  d_psi_d_SG_D_1_block : Subsystem
  d_psi_fd_SG_D_1_block : Subsystem
  d_psi_gq_SG_D_1_block : Subsystem
  d_psi_kq_SG_D_1_block : Subsystem
  d_psi_q_SG_D_1_block : Subsystem
  d_theta_SG_D_1_block : Subsystem
  d_w_SG_D_1_block : Subsystem
  i_d_SG_D_1_block : Subsystem
  i_q_SG_D_1_block : Subsystem
  psi_1d_SG_D_1 : Integrator  InitialCondition=0.7866048970248269
  psi_d_SG_D_1 : Integrator  InitialCondition=0.7492658124363175
  psi_fd_SG_D_1 : Integrator  InitialCondition=0.9747938833509144
  psi_gq_SG_D_1 : Integrator  InitialCondition=0.40843679854706383
  psi_kq_SG_D_1 : Integrator  InitialCondition=-0.6381824977297872
  psi_q_SG_D_1 : Integrator  InitialCondition=-0.6637097976389787
  theta_SG_D_1 : Integrator  InitialCondition=0.7246818835631345
  theta_SG_D_1_out_block : Subsystem
  w_SG_D_1 : Integrator  InitialCondition=376.99111843077515
  w_SG_D_1_out_block : Subsystem
  i_d_SG_D_1 : Outport
  i_q_SG_D_1 : Outport  Port=2
  T_e_SG_D_1 : Outport  Port=3
  w_SG_D_1_out : Outport  Port=4
  theta_SG_D_1_out : Outport  Port=5
  wires:
  d_theta_SG_D_1_block/1(Blockout_d_theta_SG_D_1_9a995) -> theta_SG_D_1/1
  d_Px_1_SG_D_1_block/1(Blockout_d_Px_1_SG_D_1_0803c) -> Px_1_SG_D_1/1
  V_f_SG_D_1/1 -> d_V_f_SG_D_1_block/14(State_V_f_SG_D_1_97a45), d_E_fd_SG_D_1_block/2(State_V_f_SG_D_1_c71a3)
  psi_kq_SG_D_1/1 -> i_d_SG_D_1_block/2(State_psi_kq_SG_D_1_6f9a9), i_q_SG_D_1_block/2(State_psi_kq_SG_D_1_97f5f), d_w_SG_D_1_block/5(State_psi_kq_SG_D_1_51584), T_e_SG_D_1_block/3(State_psi_kq_SG_D_1_8a639), d_V_f_SG_D_1_block/10(State_psi_kq_SG_D_1_f306c), d_psi_gq_SG_D_1_block/8(State_psi_kq_SG_D_1_b0870), d_psi_gq_SG_D_1_block/5(State_psi_kq_SG_D_1_4c797), d_psi_gq_SG_D_1_block/3(State_psi_kq_SG_D_1_1f92e), d_psi_q_SG_D_1_block/2(State_psi_kq_SG_D_1_d4ed3), d_psi_kq_SG_D_1_block/4(State_psi_kq_SG_D_1_1396d), d_psi_kq_SG_D_1_block/2(State_psi_kq_SG_D_1_02235)
  w_SG_D_1_out_block/1(Blockout_w_SG_D_1_out_45494) -> w_SG_D_1_out/1
  w_SG_D_1/1 -> d_w_SG_D_1_block/1(State_w_SG_D_1_21472), d_theta_SG_D_1_block/1(State_w_SG_D_1_c5d1e), d_T_m_SG_D_1_block/1(State_w_SG_D_1_70e26), d_Px_2_SG_D_1_block/4(State_w_SG_D_1_a8905), d_V_f_SG_D_1_block/13(State_w_SG_D_1_b3f74), d_V_f_SG_D_1_block/8(State_w_SG_D_1_95a28), d_psi_q_SG_D_1_block/9(State_w_SG_D_1_a0845), d_Px_3_SG_D_1_block/6(State_w_SG_D_1_69e87), d_psi_d_SG_D_1_block/9(State_w_SG_D_1_d7dd0), w_SG_D_1_out_block/1(State_w_SG_D_1_3e49a), d_Px_1_SG_D_1_block/2(State_w_SG_D_1_e3c6b)
  d_Px_3_SG_D_1_block/1(Blockout_d_Px_3_SG_D_1_7824f) -> Px_3_SG_D_1/1
  d_Px_2_SG_D_1_block/1(Blockout_d_Px_2_SG_D_1_d0c06) -> Px_2_SG_D_1/1
  d_T_m_SG_D_1_block/1(Blockout_d_T_m_SG_D_1_fd2e1) -> T_m_SG_D_1/1
  psi_q_SG_D_1/1 -> i_d_SG_D_1_block/3(State_psi_q_SG_D_1_9d632), i_q_SG_D_1_block/3(State_psi_q_SG_D_1_fdadd), d_w_SG_D_1_block/7(State_psi_q_SG_D_1_7fdb2), d_w_SG_D_1_block/6(State_psi_q_SG_D_1_9cbd2), d_psi_d_SG_D_1_block/8(State_psi_q_SG_D_1_b67fc), T_e_SG_D_1_block/5(State_psi_q_SG_D_1_4af3a), T_e_SG_D_1_block/4(State_psi_q_SG_D_1_d45ef), d_V_f_SG_D_1_block/11(State_psi_q_SG_D_1_520b8), d_V_f_SG_D_1_block/7(State_psi_q_SG_D_1_3613a), d_psi_gq_SG_D_1_block/6(State_psi_q_SG_D_1_eafc3), d_psi_gq_SG_D_1_block/9(State_psi_q_SG_D_1_b97dd), d_psi_q_SG_D_1_block/3(State_psi_q_SG_D_1_8f107), d_psi_kq_SG_D_1_block/5(State_psi_q_SG_D_1_e7314)
  v_d_SG_D_1/1 -> d_psi_d_SG_D_1_block/4(Input_v_d_SG_D_1_cbb22), d_psi_q_SG_D_1_block/4(Input_v_d_SG_D_1_e85f7)
  v_q_SG_D_1/1 -> d_psi_d_SG_D_1_block/6(Input_v_q_SG_D_1_0bc0c), d_psi_q_SG_D_1_block/6(Input_v_q_SG_D_1_46a58)
  Px_1_SG_D_1/1 -> d_Px_2_SG_D_1_block/2(State_Px_1_SG_D_1_2200d), d_Px_2_SG_D_1_block/3(State_Px_1_SG_D_1_dd625), d_Px_3_SG_D_1_block/4(State_Px_1_SG_D_1_61697), d_Px_3_SG_D_1_block/5(State_Px_1_SG_D_1_5b4a8), d_Px_1_SG_D_1_block/1(State_Px_1_SG_D_1_eded1)
  Px_2_SG_D_1/1 -> d_Px_3_SG_D_1_block/2(State_Px_2_SG_D_1_b59b6), d_Px_3_SG_D_1_block/3(State_Px_2_SG_D_1_6cb1b), d_Px_2_SG_D_1_block/1(State_Px_2_SG_D_1_70d74)
  T_m_SG_D_1/1 -> d_T_m_SG_D_1_block/2(State_T_m_SG_D_1_20e91), d_w_SG_D_1_block/2(State_T_m_SG_D_1_4c7a9)
  theta_SG_D_1/1 -> i_q_SG_D_1_block/4(State_theta_SG_D_1_3c1fa), i_q_SG_D_1_block/8(State_theta_SG_D_1_71fb6), i_d_SG_D_1_block/8(State_theta_SG_D_1_13345), i_d_SG_D_1_block/4(State_theta_SG_D_1_64896), d_psi_d_SG_D_1_block/7(State_theta_SG_D_1_d58f8), theta_SG_D_1_out_block/1(State_theta_SG_D_1_b223f), d_psi_q_SG_D_1_block/7(State_theta_SG_D_1_fcbfe), d_psi_q_SG_D_1_block/5(State_theta_SG_D_1_b63a1), d_psi_d_SG_D_1_block/5(State_theta_SG_D_1_f5fac)
  d_E_fd_SG_D_1_block/1(Blockout_d_E_fd_SG_D_1_f98a0) -> E_fd_SG_D_1/1
  psi_1d_SG_D_1/1 -> d_V_f_SG_D_1_block/4(State_psi_1d_SG_D_1_23908), T_e_SG_D_1_block/6(State_psi_1d_SG_D_1_4a7e6), d_psi_d_SG_D_1_block/1(State_psi_1d_SG_D_1_de078), d_psi_fd_SG_D_1_block/3(State_psi_1d_SG_D_1_0730e), d_psi_fd_SG_D_1_block/5(State_psi_1d_SG_D_1_2a034), i_q_SG_D_1_block/5(State_psi_1d_SG_D_1_7b40d), d_psi_fd_SG_D_1_block/8(State_psi_1d_SG_D_1_9f63d), d_psi_1d_SG_D_1_block/1(State_psi_1d_SG_D_1_47d5b), d_psi_1d_SG_D_1_block/3(State_psi_1d_SG_D_1_e9060), i_d_SG_D_1_block/5(State_psi_1d_SG_D_1_fc20b), d_w_SG_D_1_block/8(State_psi_1d_SG_D_1_2a3ef)
  psi_fd_SG_D_1/1 -> d_psi_fd_SG_D_1_block/2(State_psi_fd_SG_D_1_79850), d_psi_fd_SG_D_1_block/4(State_psi_fd_SG_D_1_98030), d_psi_fd_SG_D_1_block/10(State_psi_fd_SG_D_1_c1052), d_V_f_SG_D_1_block/6(State_psi_fd_SG_D_1_1b47f), T_e_SG_D_1_block/8(State_psi_fd_SG_D_1_9746c), d_psi_d_SG_D_1_block/3(State_psi_fd_SG_D_1_530eb), d_w_SG_D_1_block/10(State_psi_fd_SG_D_1_000fa), i_d_SG_D_1_block/7(State_psi_fd_SG_D_1_adb2f), i_q_SG_D_1_block/7(State_psi_fd_SG_D_1_9fe64), d_psi_1d_SG_D_1_block/2(State_psi_fd_SG_D_1_d2d5e), d_psi_1d_SG_D_1_block/5(State_psi_fd_SG_D_1_3a491), d_psi_fd_SG_D_1_block/7(State_psi_fd_SG_D_1_07c17)
  psi_gq_SG_D_1/1 -> d_psi_gq_SG_D_1_block/1(State_psi_gq_SG_D_1_fdbdc), d_psi_gq_SG_D_1_block/2(State_psi_gq_SG_D_1_7449f), d_psi_gq_SG_D_1_block/4(State_psi_gq_SG_D_1_31bfb), d_psi_kq_SG_D_1_block/1(State_psi_gq_SG_D_1_20359), d_psi_kq_SG_D_1_block/3(State_psi_gq_SG_D_1_5b14b), d_psi_gq_SG_D_1_block/7(State_psi_gq_SG_D_1_1e559), d_V_f_SG_D_1_block/9(State_psi_gq_SG_D_1_8f54b), d_psi_q_SG_D_1_block/1(State_psi_gq_SG_D_1_e06cf), T_e_SG_D_1_block/2(State_psi_gq_SG_D_1_ac02c), d_w_SG_D_1_block/4(State_psi_gq_SG_D_1_60a7b), i_d_SG_D_1_block/1(State_psi_gq_SG_D_1_5e903), i_q_SG_D_1_block/1(State_psi_gq_SG_D_1_092c5)
  psi_d_SG_D_1/1 -> d_psi_d_SG_D_1_block/2(State_psi_d_SG_D_1_bbc2d), d_w_SG_D_1_block/3(State_psi_d_SG_D_1_accda), d_w_SG_D_1_block/9(State_psi_d_SG_D_1_c53d4), i_d_SG_D_1_block/6(State_psi_d_SG_D_1_e0cb1), d_psi_fd_SG_D_1_block/9(State_psi_d_SG_D_1_1e4ac), d_V_f_SG_D_1_block/5(State_psi_d_SG_D_1_eacd9), d_psi_q_SG_D_1_block/8(State_psi_d_SG_D_1_9ece2), d_V_f_SG_D_1_block/12(State_psi_d_SG_D_1_61738), T_e_SG_D_1_block/1(State_psi_d_SG_D_1_af15c), T_e_SG_D_1_block/7(State_psi_d_SG_D_1_25ba3), d_psi_fd_SG_D_1_block/6(State_psi_d_SG_D_1_35525), d_psi_1d_SG_D_1_block/4(State_psi_d_SG_D_1_5aef1), i_q_SG_D_1_block/6(State_psi_d_SG_D_1_0e386)
  d_psi_kq_SG_D_1_block/1(Blockout_d_psi_kq_SG_D_1_1846f) -> psi_kq_SG_D_1/1
  d_psi_q_SG_D_1_block/1(Blockout_d_psi_q_SG_D_1_00fdb) -> psi_q_SG_D_1/1
  d_psi_gq_SG_D_1_block/1(Blockout_d_psi_gq_SG_D_1_83fa8) -> psi_gq_SG_D_1/1
  d_V_f_SG_D_1_block/1(Blockout_d_V_f_SG_D_1_28a77) -> V_f_SG_D_1/1
  T_e_SG_D_1_block/1(Blockout_T_e_SG_D_1_d526f) -> T_e_SG_D_1/1
  d_R_f_SG_D_1_block/1(Blockout_d_R_f_SG_D_1_964e4) -> R_f_SG_D_1/1
  d_psi_d_SG_D_1_block/1(Blockout_d_psi_d_SG_D_1_d98e5) -> psi_d_SG_D_1/1
  d_w_SG_D_1_block/1(Blockout_d_w_SG_D_1_60389) -> w_SG_D_1/1
  i_d_SG_D_1_block/1(Blockout_i_d_SG_D_1_272fd) -> i_d_SG_D_1/1
  i_q_SG_D_1_block/1(Blockout_i_q_SG_D_1_cd846) -> i_q_SG_D_1/1
  d_psi_1d_SG_D_1_block/1(Blockout_d_psi_1d_SG_D_1_60e48) -> psi_1d_SG_D_1/1
  theta_SG_D_1_out_block/1(Blockout_theta_SG_D_1_out_ac5bf) -> theta_SG_D_1_out/1
  R_f_SG_D_1/1 -> d_V_f_SG_D_1_block/2(State_R_f_SG_D_1_3a49b), d_R_f_SG_D_1_block/2(State_R_f_SG_D_1_ca3b1)
  Px_3_SG_D_1/1 -> d_V_f_SG_D_1_block/3(State_Px_3_SG_D_1_f266c), d_Px_3_SG_D_1_block/1(State_Px_3_SG_D_1_38fc8)
  E_fd_SG_D_1/1 -> d_V_f_SG_D_1_block/1(State_E_fd_SG_D_1_72ce1), d_R_f_SG_D_1_block/1(State_E_fd_SG_D_1_9aa07), d_E_fd_SG_D_1_block/1(State_E_fd_SG_D_1_dda34), d_psi_fd_SG_D_1_block/1(State_E_fd_SG_D_1_8116a)
  d_psi_fd_SG_D_1_block/1(Blockout_d_psi_fd_SG_D_1_0a2c3) -> psi_fd_SG_D_1/1
